simulink model "Shower_model"  (R2020b)
settings: Solver=FixedStepAuto  StartTime=0.0  StopTime=10  RelTol=1e-3
model workspace (MAT data in the model file):
  Idx_1 = [1 1 1 2 2 2 3 3 3]
  Idx_2 = [4 5 6 4 5 6 4 5 6]
  time = [0 0.0625 0.125 0.1875 0.25 0.3125 0.375 0.4375 0.5]
libraries: dspmtrx3 x20, simulink x2
settings Model: ParameterArgumentNames=Idx_1,Idx_2,time  OrderedModelArguments=off  Creator=Deept  LastModifiedBy=Deept
settings DebuggingCC: UnderSpecifiedDimensionMsg=warning

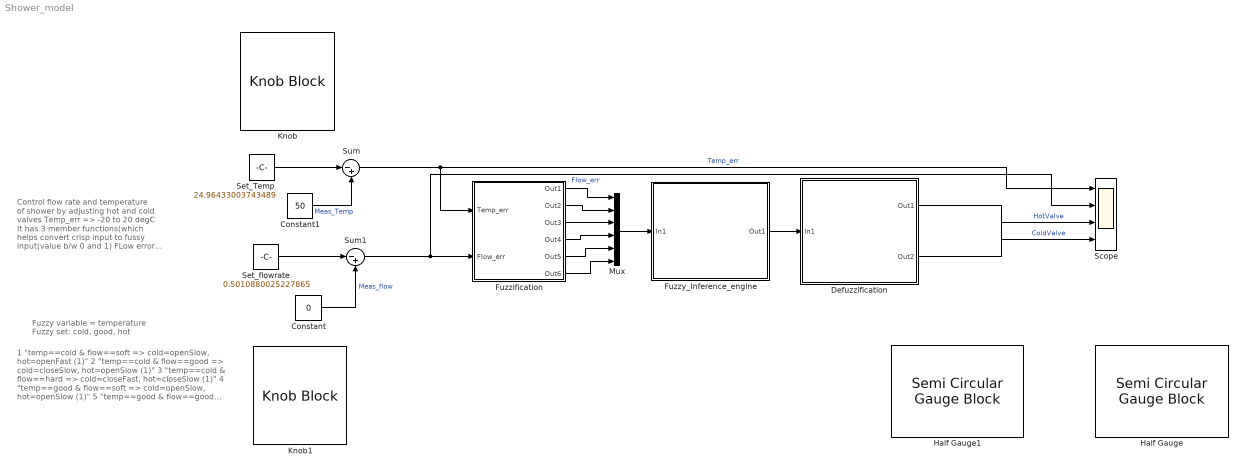
== system Shower_model ==
  note: Fuzzy variable = temperature
      | Fuzzy set: cold, good, hot
  note: 1 "temp==cold & flow==soft => cold=openSlow, hot=openFast (1)"
      | 2 "temp==cold & flow==good => cold=closeSlow, hot=openSlow (1)"
      | 3 "temp==cold & flow==hard => cold=closeFast, hot=closeSlow (1)"
      | 4 "temp==good & flow==soft => cold=openSlow, hot=openSlow (1)"
      | 5 "temp==good & flow==good => cold=steady, hot=steady (1)"
      | 6 "temp==good & flow==hard => cold=closeSlow, hot=closeSlow (1)"
      | 7 "temp==hot & flow==soft => cold=openFast, hot=openSlow (1)"
      | 8 "temp==hot & flow==good => cold=openSlow, hot=closeSlow (1)"
      | 9 "temp==hot & flow==hard => cold=closeSlow, hot=closeFast (1)"
  note: Control flow rate and temperature of shower by adjusting hot and cold valves
      |
      | Temp_err => -20 to 20 degC
      | It has 3 member functions(which helps convert crisp input to fussy input(value b/w 0 and 1)
      | FLow error => -1 to 1
  Constant : Constant  Value=0
  Constant1 : Constant  Value=50
  Defuzzification : Subsystem
  Fuzzification : Subsystem
  Fuzzy_Inference_engine : Subsystem
  Half Gauge : SemiCircularGaugeBlock  LabelPosition=Bottom  ScaleMin=-1  ScaleMax=1
  Half Gauge1 : SemiCircularGaugeBlock  LabelPosition=Bottom  ScaleMin=-1  ScaleMax=1
  Knob : KnobBlock  LabelPosition=Bottom  ScaleMin=20  ScaleMax=30
  Knob1 : KnobBlock  LabelPosition=Bottom  ScaleMax=1
  Mux : Mux  Inputs=6
  Scope : Scope  NumInputPorts=4
  Set_Temp : Constant  Value=24.96433003743489
  Set_flowrate : Constant  Value=0.5010880025227865
  Sum : Sum  Inputs=|-+
  Sum1 : Sum  Inputs=|-+
  wires:
  Set_Temp/1 -> Sum/1
  Set_flowrate/1 -> Sum1/1
  Constant1/1 -> Sum/2  "Meas_Temp"
  Constant/1 -> Sum1/2  "Meas_flow"
  Mux/1 -> Fuzzy_Inference_engine/1(In1)
  Sum/1 -> Fuzzification/1(Temp_err), Scope/1  "Temp_err"
  Sum1/1 -> Fuzzification/2(Flow_err), Scope/2  "Flow_err"
  Fuzzification/1(Out1) -> Mux/1
  Fuzzification/2(Out2) -> Mux/2
  Fuzzification/3(Out3) -> Mux/3
  Fuzzification/4(Out4) -> Mux/4
  Fuzzification/5(Out5) -> Mux/5
  Fuzzification/6(Out6) -> Mux/6
  Fuzzy_Inference_engine/1(Out1) -> Defuzzification/1(In1)
  Defuzzification/1(Out1) -> Scope/4  "ColdValve"
  Defuzzification/2(Out2) -> Scope/3  "HotValve"

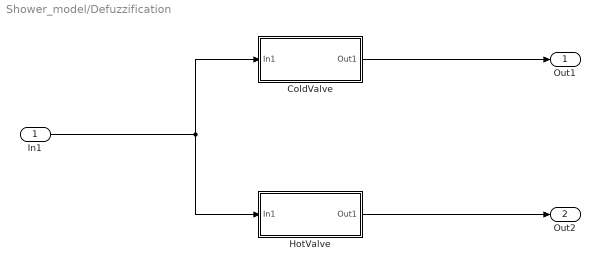
== system Shower_model/Defuzzification ==
  In1 : Inport
  ColdValve : Subsystem
  HotValve : Subsystem
  Out1 : Outport
  Out2 : Outport  Port=2
  wires:
  In1/1 -> ColdValve/1(In1), HotValve/1(In1)
  ColdValve/1(Out1) -> Out1/1
  HotValve/1(Out1) -> Out2/1

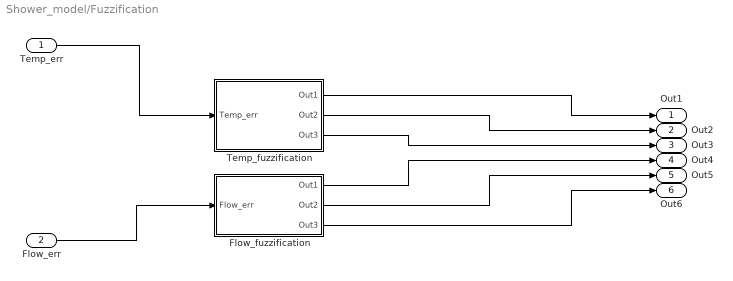
== system Shower_model/Fuzzification ==
  Temp_err : Inport
  Flow_err : Inport  Port=2
  Flow_fuzzification : Subsystem
  Temp_fuzzification : Subsystem
  Out1 : Outport
  Out2 : Outport  Port=2
  Out3 : Outport  Port=3
  Out4 : Outport  Port=4
  Out5 : Outport  Port=5
  Out6 : Outport  Port=6
  wires:
  Temp_err/1 -> Temp_fuzzification/1(Temp_err)
  Flow_fuzzification/1(Out1) -> Out4/1
  Flow_err/1 -> Flow_fuzzification/1(Flow_err)
  Flow_fuzzification/3(Out3) -> Out6/1
  Flow_fuzzification/2(Out2) -> Out5/1
  Temp_fuzzification/1(Out1) -> Out1/1
  Temp_fuzzification/3(Out3) -> Out3/1
  Temp_fuzzification/2(Out2) -> Out2/1

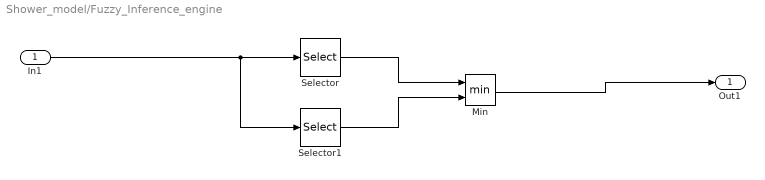
== system Shower_model/Fuzzy_Inference_engine ==
  In1 : Inport
  Min : MinMax  Inputs=2
  Selector : Selector  InputPortWidth=6  IndexOptions=Index vector (dialog)  Indices=idx_1  OutputSizes=1
  Selector1 : Selector  InputPortWidth=6  IndexOptions=Index vector (dialog)  Indices=idx_2  OutputSizes=1
  Out1 : Outport
  wires:
  Min/1 -> Out1/1
  Selector/1 -> Min/1
  Selector1/1 -> Min/2
  In1/1 -> Selector1/1, Selector/1

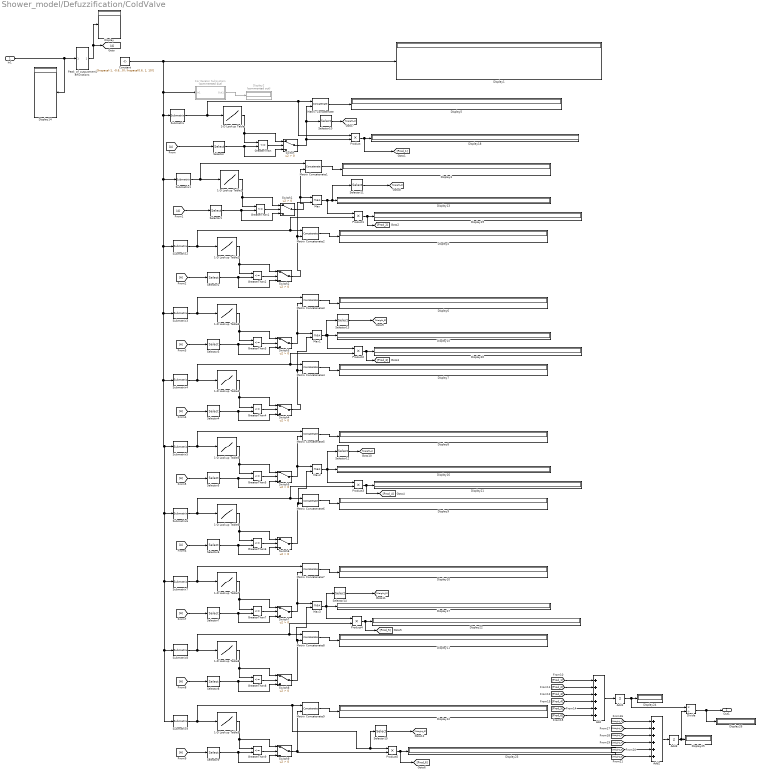
== system Shower_model/Defuzzification/ColdValve ==
  In1 : Inport
  1-D Lookup Table : Lookup_n-D  NumberOfTableDimensions=1  BreakpointsForDimension1=linspace(-1, -0.6, 10)  Table=(linspace(-1, -0.6, 10) + 1) / 0.4  InternalRulePriority=Speed  RndMeth=Simplest  InputSameDT=on
  1-D Lookup Table1 : Lookup_n-D  NumberOfTableDimensions=1  BreakpointsForDimension1=linspace(-0.6, -0.3, 10)  Table=-(linspace(-0.6, -0.3, 10) + 0.3) / 0.3  InternalRulePriority=Speed  RndMeth=Simplest  InputSameDT=on
  1-D Lookup Table2 : Lookup_n-D  NumberOfTableDimensions=1  BreakpointsForDimension1=linspace(-0.6, -0.3, 10)  Table=(linspace(-0.6, -0.3, 10) + 0.6) / 0.3  InternalRulePriority=Speed  RndMeth=Simplest  InputSameDT=on
  1-D Lookup Table3 : Lookup_n-D  NumberOfTableDimensions=1  BreakpointsForDimension1=linspace(-0.3, 0, 10)  Table=-linspace(-0.3, 0, 10) / 0.3  InternalRulePriority=Speed  RndMeth=Simplest  InputSameDT=on
  1-D Lookup Table4 : Lookup_n-D  NumberOfTableDimensions=1  BreakpointsForDimension1=linspace(-0.3, 0, 10)  Table=(linspace(-0.3, 0, 10) + 0.3) / 0.3  InternalRulePriority=Speed  RndMeth=Simplest  InputSameDT=on
  1-D Lookup Table5 : Lookup_n-D  NumberOfTableDimensions=1  BreakpointsForDimension1=linspace(0, 0.3, 10)  Table=-(linspace(0, 0.3, 10) - 0.3) / 0.3  InternalRulePriority=Speed  RndMeth=Simplest  InputSameDT=on
  1-D Lookup Table6 : Lookup_n-D  NumberOfTableDimensions=1  BreakpointsForDimension1=linspace(0, 0.3, 10)  Table=linspace(0, 0.3, 10) / 0.3  InternalRulePriority=Speed  RndMeth=Simplest  InputSameDT=on
  1-D Lookup Table7 : Lookup_n-D  NumberOfTableDimensions=1  BreakpointsForDimension1=linspace(0.3, 0.6, 10)  Table=-(linspace(0.3, 0.6, 10) - 0.6) / 0.3  InternalRulePriority=Speed  RndMeth=Simplest  InputSameDT=on
  1-D Lookup Table8 : Lookup_n-D  NumberOfTableDimensions=1  BreakpointsForDimension1=linspace(0.3, 0.6, 10)  Table=(linspace(0.3, 0.6, 10) - 0.3) / 0.3  InternalRulePriority=Speed  RndMeth=Simplest  InputSameDT=on
  1-D Lookup Table9 : Lookup_n-D  NumberOfTableDimensions=1  BreakpointsForDimension1=linspace(0.6, 1, 10)  Table=-(linspace(0.6, 1, 10) - 1) / 0.4  InternalRulePriority=Speed  RndMeth=Simplest  InputSameDT=on
  Add : Sum  Inputs=++++++
  Add1 : Sum  Inputs=+
  Add2 : Sum  Inputs=++++++
  Add3 : Sum  Inputs=+
  Constant : Constant  Value=[linspace(-1, -0.6, 10); linspace(-0.6, -0.3, 10); linspace(-0.3, 0, 10); linspace(0, 0.3, 10); linspace(0.3, 0.6, 10); linspace(0.6, 1, 10)]
  Display{,1,3..26} (26 alike) : Display
  Display2 : Display  Commented=on
  Divide : Product  Inputs=*/
  For Iterator Subsystem : Subsystem  Commented=on  TreatAsAtomicUnit=on
  GreaterThan{,1..9} (10 alike) : RelationalOperator  Operator=<=  OutDataTypeStr=boolean  RndMeth=Simplest
  Matrix Concatenate{,1..9} (10 alike) : Concatenate  Mode=Multidimensional array  ConcatenateDimension=2
  Max{,1..3} (4 alike) : MinMax  Function=max  Inputs=2
  Peak_of_outputmemberfunctions : Subsystem
  Product{,1..5} (6 alike) : Product
  Selector : Selector  InputPortWidth=5  IndexOptions=Index vector (dialog)  Indices=1  OutputSizes=1
  Selector1 : Selector  InputPortWidth=5  IndexOptions=Index vector (dialog)  Indices=1  OutputSizes=1
  Selector{10..15} (6 alike) : Selector  InputPortWidth=10  IndexOptions=Index vector (dialog)  Indices=[1:9]  OutputSizes=1
  Selector2 : Selector  InputPortWidth=5  IndexOptions=Index vector (dialog)  Indices=2  OutputSizes=1
  Selector3 : Selector  InputPortWidth=5  IndexOptions=Index vector (dialog)  Indices=2  OutputSizes=1
  Selector4 : Selector  InputPortWidth=5  IndexOptions=Index vector (dialog)  Indices=3  OutputSizes=1
  Selector5 : Selector  InputPortWidth=5  IndexOptions=Index vector (dialog)  Indices=3  OutputSizes=1
  Selector6 : Selector  InputPortWidth=5  IndexOptions=Index vector (dialog)  Indices=4  OutputSizes=1
  Selector7 : Selector  InputPortWidth=5  IndexOptions=Index vector (dialog)  Indices=4  OutputSizes=1
  Selector8 : Selector  InputPortWidth=5  IndexOptions=Index vector (dialog)  Indices=5  OutputSizes=1
  Selector9 : Selector  InputPortWidth=5  IndexOptions=Index vector (dialog)  Indices=5  OutputSizes=1
  Submatrix : dspmtrx3/Submatrix  RowSpan=Range of rows  RowStartMode=Index  RowStartIndex=1  RowEndMode=Index  RowEndIndex=1  ColSpan=All columns  ColStartMode=First  ColStartIndex=1  ColEndMode=Last  ColEndIndex=1
  Submatrix1 : dspmtrx3/Submatrix  RowSpan=Range of rows  RowStartMode=Index  RowStartIndex=2  RowEndMode=Index  RowEndIndex=2  ColSpan=All columns  ColStartMode=First  ColStartIndex=1  ColEndMode=Last  ColEndIndex=1
  Submatrix2 : dspmtrx3/Submatrix  RowSpan=Range of rows  RowStartMode=Index  RowStartIndex=2  RowEndMode=Index  RowEndIndex=2  ColSpan=All columns  ColStartMode=First  ColStartIndex=1  ColEndMode=Last  ColEndIndex=1
  Submatrix3 : dspmtrx3/Submatrix  RowSpan=Range of rows  RowStartMode=Index  RowStartIndex=3  RowEndMode=Index  RowEndIndex=3  ColSpan=All columns  ColStartMode=First  ColStartIndex=1  ColEndMode=Last  ColEndIndex=1
  Submatrix4 : dspmtrx3/Submatrix  RowSpan=Range of rows  RowStartMode=Index  RowStartIndex=3  RowEndMode=Index  RowEndIndex=3  ColSpan=All columns  ColStartMode=First  ColStartIndex=1  ColEndMode=Last  ColEndIndex=1
  Submatrix5 : dspmtrx3/Submatrix  RowSpan=Range of rows  RowStartMode=Index  RowStartIndex=4  RowEndMode=Index  RowEndIndex=4  ColSpan=All columns  ColStartMode=First  ColStartIndex=1  ColEndMode=Last  ColEndIndex=1
  Submatrix6 : dspmtrx3/Submatrix  RowSpan=Range of rows  RowStartMode=Index  RowStartIndex=4  RowEndMode=Index  RowEndIndex=4  ColSpan=All columns  ColStartMode=First  ColStartIndex=1  ColEndMode=Last  ColEndIndex=1
  Submatrix7 : dspmtrx3/Submatrix  RowSpan=Range of rows  RowStartMode=Index  RowStartIndex=5  RowEndMode=Index  RowEndIndex=5  ColSpan=All columns  ColStartMode=First  ColStartIndex=1  ColEndMode=Last  ColEndIndex=1
  Submatrix8 : dspmtrx3/Submatrix  RowSpan=Range of rows  RowStartMode=Index  RowStartIndex=5  RowEndMode=Index  RowEndIndex=5  ColSpan=All columns  ColStartMode=First  ColStartIndex=1  ColEndMode=Last  ColEndIndex=1
  Submatrix9 : dspmtrx3/Submatrix  RowSpan=Range of rows  RowStartMode=Index  RowStartIndex=6  RowEndMode=Index  RowEndIndex=6  ColSpan=All columns  ColStartMode=First  ColStartIndex=1  ColEndMode=Last  ColEndIndex=1
  Switch{,1..9} (10 alike) : Switch  Criteria=u2 > Threshold
  Out1 : Outport
  wires:
  In1/1 -> Display14/1, Peak_of_outputmemberfunctions/1(In1)
  Peak_of_outputmemberfunctions/1(Out1) -> [A], Display/1
  For Iterator Subsystem/1(Out1) -> Display2/1
  1-D Lookup Table/1 -> Switch/1, GreaterThan/1
  [A] -> Selector/1
  GreaterThan/1 -> Switch/2
  Selector/1 -> Switch/3, GreaterThan/2
  GreaterThan1/1 -> Switch1/2
  Selector1/1 -> Switch1/3, GreaterThan1/2
  [A] -> Selector1/1
  1-D Lookup Table1/1 -> Switch1/1, GreaterThan1/1
  Switch/1 -> Product/2, Selector10/1, Matrix Concatenate/2
  Matrix Concatenate/1 -> Display5/1
  Submatrix1/1 -> Matrix Concatenate1/1, 1-D Lookup Table1/1
  Switch1/1 -> Matrix Concatenate1/2, Max/1
  Matrix Concatenate1/1 -> Display3/1
  [A] -> Selector2/1
  Switch2/1 -> Max/2, Matrix Concatenate2/2
  GreaterThan2/1 -> Switch2/2
  1-D Lookup Table2/1 -> Switch2/1, GreaterThan2/1
  Selector2/1 -> Switch2/3, GreaterThan2/2
  1-D Lookup Table3/1 -> Switch3/1, GreaterThan3/1
  GreaterThan3/1 -> Switch3/2
  [A] -> Selector3/1
  Selector3/1 -> Switch3/3, GreaterThan3/2
  Matrix Concatenate3/1 -> Display6/1
  Submatrix3/1 -> Matrix Concatenate3/1, 1-D Lookup Table3/1
  Matrix Concatenate4/1 -> Display7/1
  Selector4/1 -> Switch4/3, GreaterThan4/2
  [A] -> Selector4/1
  1-D Lookup Table4/1 -> Switch4/1, GreaterThan4/1
  GreaterThan4/1 -> Switch4/2
  GreaterThan5/1 -> Switch5/2
  Submatrix5/1 -> Matrix Concatenate5/1, 1-D Lookup Table5/1
  1-D Lookup Table5/1 -> Switch5/1, GreaterThan5/1
  Matrix Concatenate5/1 -> Display8/1
  Selector5/1 -> Switch5/3, GreaterThan5/2
  [A] -> Selector5/1
  Matrix Concatenate6/1 -> Display9/1
  [A] -> Selector6/1
  Selector6/1 -> Switch6/3, GreaterThan6/2
  1-D Lookup Table6/1 -> Switch6/1, GreaterThan6/1
  GreaterThan6/1 -> Switch6/2
  1-D Lookup Table7/1 -> Switch7/1, GreaterThan7/1
  GreaterThan7/1 -> Switch7/2
  Submatrix7/1 -> Matrix Concatenate7/1, 1-D Lookup Table7/1
  Selector7/1 -> Switch7/3, GreaterThan7/2
  [A] -> Selector7/1
  Matrix Concatenate7/1 -> Display10/1
  Selector8/1 -> Switch8/3, GreaterThan8/2
  [A] -> Selector8/1
  Matrix Concatenate8/1 -> Display11/1
  GreaterThan8/1 -> Switch8/2
  1-D Lookup Table8/1 -> Switch8/1, GreaterThan8/1
  Constant/1 -> For Iterator Subsystem/1(In1), Submatrix2/1, Submatrix9/1, Submatrix8/1, Submatrix7/1, Submatrix6/1, Submatrix5/1, Submatrix4/1, Submatrix3/1, Submatrix1/1, Submatrix/1, Display1/1
  Selector9/1 -> Switch9/3, GreaterThan9/2
  1-D Lookup Table9/1 -> Switch9/1, GreaterThan9/1
  GreaterThan9/1 -> Switch9/2
  [A] -> Selector9/1
  Matrix Concatenate9/1 -> Display12/1
  Matrix Concatenate2/1 -> Display4/1
  Switch3/1 -> Max1/1, Matrix Concatenate3/2
  Switch4/1 -> Max1/2, Matrix Concatenate4/2
  Switch5/1 -> Max2/1, Matrix Concatenate5/2
  Switch6/1 -> Max2/2, Matrix Concatenate6/2
  Switch8/1 -> Matrix Concatenate8/2, Max3/2
  Switch7/1 -> Max3/1, Matrix Concatenate7/2
  Product/1 -> [Prod_1], Display18/1
  Submatrix2/1 -> Product1/2, Matrix Concatenate2/1, 1-D Lookup Table2/1
  Product1/1 -> [Prod_2], Display19/1
  Max/1 -> Selector11/1, Display13/1, Product1/1
  Max1/1 -> Selector13/1, Product2/1, Display15/1
  Submatrix4/1 -> Product2/2, Matrix Concatenate4/1, 1-D Lookup Table4/1
  Product2/1 -> [Prod_3], Display20/1
  Max2/1 -> Product3/1, Selector12/1, Display16/1
  Product3/1 -> [Prod_4], Display21/1
  Submatrix6/1 -> Product3/2, Matrix Concatenate6/1, 1-D Lookup Table6/1
  Max3/1 -> Selector14/1, Product4/1, Display17/1
  Product4/1 -> [Prod_5], Display22/1
  Submatrix8/1 -> Product4/2, Matrix Concatenate8/1, 1-D Lookup Table8/1
  Submatrix9/1 -> Selector15/1, Product5/1, Matrix Concatenate9/1, 1-D Lookup Table9/1
  Product5/1 -> [Prod_6], Display23/1
  Switch9/1 -> Matrix Concatenate9/2, Product5/2
  [Prod_1] -> Add/1
  [Prod_2] -> Add/2
  [Prod_3] -> Add/3
  [Prod_4] -> Add/4
  [Prod_5] -> Add/5
  [Prod_6] -> Add/6
  Add/1 -> Add1/1
  Add1/1 -> Divide/1, Display24/1
  [Weight_3] -> Add2/3
  [Weight_6] -> Add2/6
  [Weight_1] -> Add2/1
  [Weight_5] -> Add2/5
  [Weight_2] -> Add2/2
  [Weight_4] -> Add2/4
  Add2/1 -> Add3/1
  Add3/1 -> Divide/2, Display25/1
  Submatrix/1 -> Matrix Concatenate/1, Product/1, 1-D Lookup Table/1
  Selector10/1 -> [Weight_1]
  Selector11/1 -> [Weight_2]
  Selector13/1 -> [Weight_3]
  Selector12/1 -> [Weight_4]
  Selector14/1 -> [Weight_5]
  Selector15/1 -> [Weight_6]
  Divide/1 -> Out1/1, Display26/1

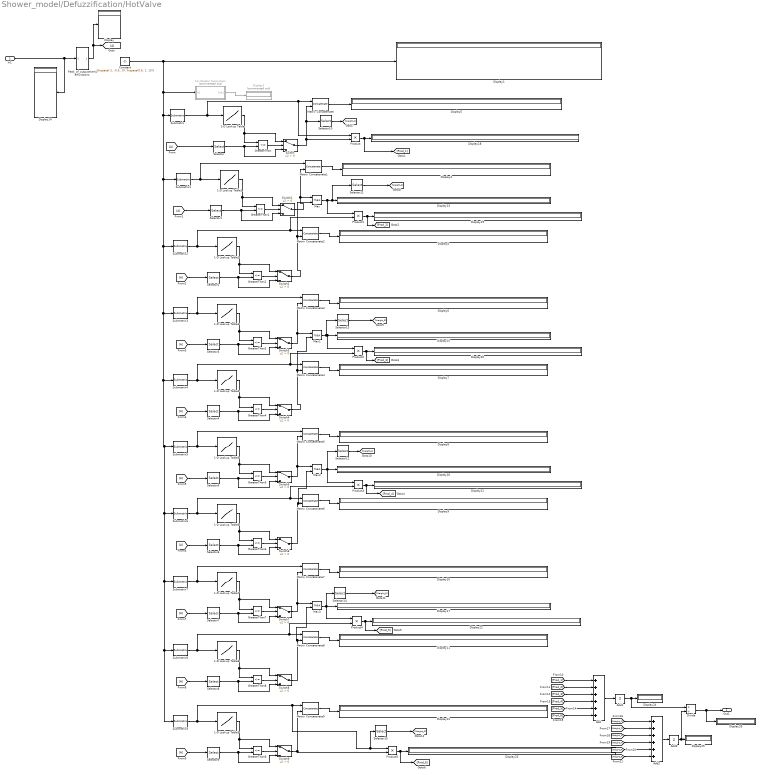
== system Shower_model/Defuzzification/HotValve ==
  In1 : Inport
  1-D Lookup Table : Lookup_n-D  NumberOfTableDimensions=1  BreakpointsForDimension1=linspace(-1, -0.6, 10)  Table=(linspace(-1, -0.6, 10) + 1) / 0.4  InternalRulePriority=Speed  RndMeth=Simplest  InputSameDT=on
  1-D Lookup Table1 : Lookup_n-D  NumberOfTableDimensions=1  BreakpointsForDimension1=linspace(-0.6, -0.3, 10)  Table=-(linspace(-0.6, -0.3, 10) + 0.3) / 0.3  InternalRulePriority=Speed  RndMeth=Simplest  InputSameDT=on
  1-D Lookup Table2 : Lookup_n-D  NumberOfTableDimensions=1  BreakpointsForDimension1=linspace(-0.6, -0.3, 10)  Table=(linspace(-0.6, -0.3, 10) + 0.6) / 0.3  InternalRulePriority=Speed  RndMeth=Simplest  InputSameDT=on
  1-D Lookup Table3 : Lookup_n-D  NumberOfTableDimensions=1  BreakpointsForDimension1=linspace(-0.3, 0, 10)  Table=-linspace(-0.3, 0, 10) / 0.3  InternalRulePriority=Speed  RndMeth=Simplest  InputSameDT=on
  1-D Lookup Table4 : Lookup_n-D  NumberOfTableDimensions=1  BreakpointsForDimension1=linspace(-0.3, 0, 10)  Table=(linspace(-0.3, 0, 10) + 0.3) / 0.3  InternalRulePriority=Speed  RndMeth=Simplest  InputSameDT=on
  1-D Lookup Table5 : Lookup_n-D  NumberOfTableDimensions=1  BreakpointsForDimension1=linspace(0, 0.3, 10)  Table=-(linspace(0, 0.3, 10) - 0.3) / 0.3  InternalRulePriority=Speed  RndMeth=Simplest  InputSameDT=on
  1-D Lookup Table6 : Lookup_n-D  NumberOfTableDimensions=1  BreakpointsForDimension1=linspace(0, 0.3, 10)  Table=linspace(0, 0.3, 10) / 0.3  InternalRulePriority=Speed  RndMeth=Simplest  InputSameDT=on
  1-D Lookup Table7 : Lookup_n-D  NumberOfTableDimensions=1  BreakpointsForDimension1=linspace(0.3, 0.6, 10)  Table=-(linspace(0.3, 0.6, 10) - 0.6) / 0.3  InternalRulePriority=Speed  RndMeth=Simplest  InputSameDT=on
  1-D Lookup Table8 : Lookup_n-D  NumberOfTableDimensions=1  BreakpointsForDimension1=linspace(0.3, 0.6, 10)  Table=(linspace(0.3, 0.6, 10) - 0.3) / 0.3  InternalRulePriority=Speed  RndMeth=Simplest  InputSameDT=on
  1-D Lookup Table9 : Lookup_n-D  NumberOfTableDimensions=1  BreakpointsForDimension1=linspace(0.6, 1, 10)  Table=-(linspace(0.6, 1, 10) - 1) / 0.4  InternalRulePriority=Speed  RndMeth=Simplest  InputSameDT=on
  Add : Sum  Inputs=++++++
  Add1 : Sum  Inputs=+
  Add2 : Sum  Inputs=++++++
  Add3 : Sum  Inputs=+
  Constant : Constant  Value=[linspace(-1, -0.6, 10); linspace(-0.6, -0.3, 10); linspace(-0.3, 0, 10); linspace(0, 0.3, 10); linspace(0.3, 0.6, 10); linspace(0.6, 1, 10)]
  Display{,1,3..26} (26 alike) : Display
  Display2 : Display  Commented=on
  Divide : Product  Inputs=*/
  For Iterator Subsystem : Subsystem  Commented=on  TreatAsAtomicUnit=on
  GreaterThan{,1..9} (10 alike) : RelationalOperator  Operator=<=  OutDataTypeStr=boolean  RndMeth=Simplest
  Matrix Concatenate{,1..9} (10 alike) : Concatenate  Mode=Multidimensional array  ConcatenateDimension=2
  Max{,1..3} (4 alike) : MinMax  Function=max  Inputs=2
  Peak_of_outputmemberfunctions : Subsystem
  Product{,1..5} (6 alike) : Product
  Selector : Selector  InputPortWidth=5  IndexOptions=Index vector (dialog)  Indices=1  OutputSizes=1
  Selector1 : Selector  InputPortWidth=5  IndexOptions=Index vector (dialog)  Indices=1  OutputSizes=1
  Selector{10..15} (6 alike) : Selector  InputPortWidth=10  IndexOptions=Index vector (dialog)  Indices=[1:9]  OutputSizes=1
  Selector2 : Selector  InputPortWidth=5  IndexOptions=Index vector (dialog)  Indices=2  OutputSizes=1
  Selector3 : Selector  InputPortWidth=5  IndexOptions=Index vector (dialog)  Indices=2  OutputSizes=1
  Selector4 : Selector  InputPortWidth=5  IndexOptions=Index vector (dialog)  Indices=3  OutputSizes=1
  Selector5 : Selector  InputPortWidth=5  IndexOptions=Index vector (dialog)  Indices=3  OutputSizes=1
  Selector6 : Selector  InputPortWidth=5  IndexOptions=Index vector (dialog)  Indices=4  OutputSizes=1
  Selector7 : Selector  InputPortWidth=5  IndexOptions=Index vector (dialog)  Indices=4  OutputSizes=1
  Selector8 : Selector  InputPortWidth=5  IndexOptions=Index vector (dialog)  Indices=5  OutputSizes=1
  Selector9 : Selector  InputPortWidth=5  IndexOptions=Index vector (dialog)  Indices=5  OutputSizes=1
  Submatrix : dspmtrx3/Submatrix  RowSpan=Range of rows  RowStartMode=Index  RowStartIndex=1  RowEndMode=Index  RowEndIndex=1  ColSpan=All columns  ColStartMode=First  ColStartIndex=1  ColEndMode=Last  ColEndIndex=1
  Submatrix1 : dspmtrx3/Submatrix  RowSpan=Range of rows  RowStartMode=Index  RowStartIndex=2  RowEndMode=Index  RowEndIndex=2  ColSpan=All columns  ColStartMode=First  ColStartIndex=1  ColEndMode=Last  ColEndIndex=1
  Submatrix2 : dspmtrx3/Submatrix  RowSpan=Range of rows  RowStartMode=Index  RowStartIndex=2  RowEndMode=Index  RowEndIndex=2  ColSpan=All columns  ColStartMode=First  ColStartIndex=1  ColEndMode=Last  ColEndIndex=1
  Submatrix3 : dspmtrx3/Submatrix  RowSpan=Range of rows  RowStartMode=Index  RowStartIndex=3  RowEndMode=Index  RowEndIndex=3  ColSpan=All columns  ColStartMode=First  ColStartIndex=1  ColEndMode=Last  ColEndIndex=1
  Submatrix4 : dspmtrx3/Submatrix  RowSpan=Range of rows  RowStartMode=Index  RowStartIndex=3  RowEndMode=Index  RowEndIndex=3  ColSpan=All columns  ColStartMode=First  ColStartIndex=1  ColEndMode=Last  ColEndIndex=1
  Submatrix5 : dspmtrx3/Submatrix  RowSpan=Range of rows  RowStartMode=Index  RowStartIndex=4  RowEndMode=Index  RowEndIndex=4  ColSpan=All columns  ColStartMode=First  ColStartIndex=1  ColEndMode=Last  ColEndIndex=1
  Submatrix6 : dspmtrx3/Submatrix  RowSpan=Range of rows  RowStartMode=Index  RowStartIndex=4  RowEndMode=Index  RowEndIndex=4  ColSpan=All columns  ColStartMode=First  ColStartIndex=1  ColEndMode=Last  ColEndIndex=1
  Submatrix7 : dspmtrx3/Submatrix  RowSpan=Range of rows  RowStartMode=Index  RowStartIndex=5  RowEndMode=Index  RowEndIndex=5  ColSpan=All columns  ColStartMode=First  ColStartIndex=1  ColEndMode=Last  ColEndIndex=1
  Submatrix8 : dspmtrx3/Submatrix  RowSpan=Range of rows  RowStartMode=Index  RowStartIndex=5  RowEndMode=Index  RowEndIndex=5  ColSpan=All columns  ColStartMode=First  ColStartIndex=1  ColEndMode=Last  ColEndIndex=1
  Submatrix9 : dspmtrx3/Submatrix  RowSpan=Range of rows  RowStartMode=Index  RowStartIndex=6  RowEndMode=Index  RowEndIndex=6  ColSpan=All columns  ColStartMode=First  ColStartIndex=1  ColEndMode=Last  ColEndIndex=1
  Switch{,1..9} (10 alike) : Switch  Criteria=u2 > Threshold
  Out1 : Outport
  wires:
  In1/1 -> Display14/1, Peak_of_outputmemberfunctions/1(In1)
  Peak_of_outputmemberfunctions/1(Out1) -> [A], Display/1
  For Iterator Subsystem/1(Out1) -> Display2/1
  1-D Lookup Table/1 -> Switch/1, GreaterThan/1
  [A] -> Selector/1
  GreaterThan/1 -> Switch/2
  Selector/1 -> Switch/3, GreaterThan/2
  GreaterThan1/1 -> Switch1/2
  Selector1/1 -> Switch1/3, GreaterThan1/2
  [A] -> Selector1/1
  1-D Lookup Table1/1 -> Switch1/1, GreaterThan1/1
  Switch/1 -> Product/2, Selector10/1, Matrix Concatenate/2
  Matrix Concatenate/1 -> Display5/1
  Submatrix1/1 -> Matrix Concatenate1/1, 1-D Lookup Table1/1
  Switch1/1 -> Matrix Concatenate1/2, Max/1
  Matrix Concatenate1/1 -> Display3/1
  [A] -> Selector2/1
  Switch2/1 -> Max/2, Matrix Concatenate2/2
  GreaterThan2/1 -> Switch2/2
  1-D Lookup Table2/1 -> Switch2/1, GreaterThan2/1
  Selector2/1 -> Switch2/3, GreaterThan2/2
  1-D Lookup Table3/1 -> Switch3/1, GreaterThan3/1
  GreaterThan3/1 -> Switch3/2
  [A] -> Selector3/1
  Selector3/1 -> Switch3/3, GreaterThan3/2
  Matrix Concatenate3/1 -> Display6/1
  Submatrix3/1 -> Matrix Concatenate3/1, 1-D Lookup Table3/1
  Matrix Concatenate4/1 -> Display7/1
  Selector4/1 -> Switch4/3, GreaterThan4/2
  [A] -> Selector4/1
  1-D Lookup Table4/1 -> Switch4/1, GreaterThan4/1
  GreaterThan4/1 -> Switch4/2
  GreaterThan5/1 -> Switch5/2
  Submatrix5/1 -> Matrix Concatenate5/1, 1-D Lookup Table5/1
  1-D Lookup Table5/1 -> Switch5/1, GreaterThan5/1
  Matrix Concatenate5/1 -> Display8/1
  Selector5/1 -> Switch5/3, GreaterThan5/2
  [A] -> Selector5/1
  Matrix Concatenate6/1 -> Display9/1
  [A] -> Selector6/1
  Selector6/1 -> Switch6/3, GreaterThan6/2
  1-D Lookup Table6/1 -> Switch6/1, GreaterThan6/1
  GreaterThan6/1 -> Switch6/2
  1-D Lookup Table7/1 -> Switch7/1, GreaterThan7/1
  GreaterThan7/1 -> Switch7/2
  Submatrix7/1 -> Matrix Concatenate7/1, 1-D Lookup Table7/1
  Selector7/1 -> Switch7/3, GreaterThan7/2
  [A] -> Selector7/1
  Matrix Concatenate7/1 -> Display10/1
  Selector8/1 -> Switch8/3, GreaterThan8/2
  [A] -> Selector8/1
  Matrix Concatenate8/1 -> Display11/1
  GreaterThan8/1 -> Switch8/2
  1-D Lookup Table8/1 -> Switch8/1, GreaterThan8/1
  Constant/1 -> For Iterator Subsystem/1(In1), Submatrix2/1, Submatrix9/1, Submatrix8/1, Submatrix7/1, Submatrix6/1, Submatrix5/1, Submatrix4/1, Submatrix3/1, Submatrix1/1, Submatrix/1, Display1/1
  Selector9/1 -> Switch9/3, GreaterThan9/2
  1-D Lookup Table9/1 -> Switch9/1, GreaterThan9/1
  GreaterThan9/1 -> Switch9/2
  [A] -> Selector9/1
  Matrix Concatenate9/1 -> Display12/1
  Matrix Concatenate2/1 -> Display4/1
  Switch3/1 -> Max1/1, Matrix Concatenate3/2
  Switch4/1 -> Max1/2, Matrix Concatenate4/2
  Switch5/1 -> Max2/1, Matrix Concatenate5/2
  Switch6/1 -> Max2/2, Matrix Concatenate6/2
  Switch8/1 -> Matrix Concatenate8/2, Max3/2
  Switch7/1 -> Max3/1, Matrix Concatenate7/2
  Product/1 -> [Prod_1], Display18/1
  Submatrix2/1 -> Product1/2, Matrix Concatenate2/1, 1-D Lookup Table2/1
  Product1/1 -> [Prod_2], Display19/1
  Max/1 -> Selector11/1, Display13/1, Product1/1
  Max1/1 -> Selector13/1, Product2/1, Display15/1
  Submatrix4/1 -> Product2/2, Matrix Concatenate4/1, 1-D Lookup Table4/1
  Product2/1 -> [Prod_3], Display20/1
  Max2/1 -> Product3/1, Selector12/1, Display16/1
  Product3/1 -> [Prod_4], Display21/1
  Submatrix6/1 -> Product3/2, Matrix Concatenate6/1, 1-D Lookup Table6/1
  Max3/1 -> Selector14/1, Product4/1, Display17/1
  Product4/1 -> [Prod_5], Display22/1
  Submatrix8/1 -> Product4/2, Matrix Concatenate8/1, 1-D Lookup Table8/1
  Submatrix9/1 -> Selector15/1, Product5/1, Matrix Concatenate9/1, 1-D Lookup Table9/1
  Product5/1 -> [Prod_6], Display23/1
  Switch9/1 -> Matrix Concatenate9/2, Product5/2
  [Prod_1] -> Add/1
  [Prod_2] -> Add/2
  [Prod_3] -> Add/3
  [Prod_4] -> Add/4
  [Prod_5] -> Add/5
  [Prod_6] -> Add/6
  Add/1 -> Add1/1
  Add1/1 -> Divide/1, Display24/1
  [Weight_3] -> Add2/3
  [Weight_6] -> Add2/6
  [Weight_1] -> Add2/1
  [Weight_5] -> Add2/5
  [Weight_2] -> Add2/2
  [Weight_4] -> Add2/4
  Add2/1 -> Add3/1
  Add3/1 -> Divide/2, Display25/1
  Submatrix/1 -> Matrix Concatenate/1, Product/1, 1-D Lookup Table/1
  Selector10/1 -> [Weight_1]
  Selector11/1 -> [Weight_2]
  Selector13/1 -> [Weight_3]
  Selector12/1 -> [Weight_4]
  Selector14/1 -> [Weight_5]
  Selector15/1 -> [Weight_6]
  Divide/1 -> Out1/1, Display26/1

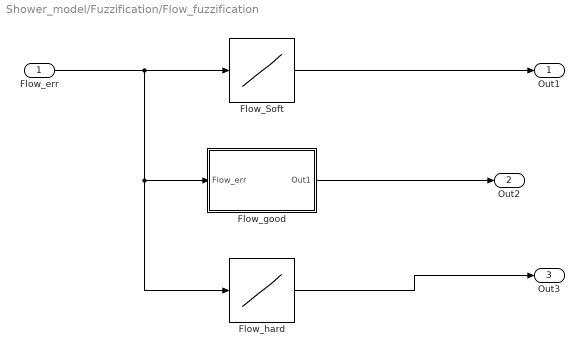
== system Shower_model/Fuzzification/Flow_fuzzification ==
  Flow_err : Inport
  Flow_Soft : Lookup_n-D  NumberOfTableDimensions=1  BreakpointsForDimension1=linspace(-0.8, 0, 10)  Table=(linspace(-0.8, 0, 10)) / (-0.8)  ExtrapMethod=Clip  InternalRulePriority=Speed  RndMeth=Simplest  InputSameDT=on
  Flow_good : Subsystem
  Flow_hard : Lookup_n-D  NumberOfTableDimensions=1  BreakpointsForDimension1=linspace(0, 0.8, 10)  Table=linspace(0, 0.8, 10) / 0.8  ExtrapMethod=Clip  InternalRulePriority=Speed  RndMeth=Simplest  InputSameDT=on
  Out1 : Outport
  Out2 : Outport  Port=2
  Out3 : Outport  Port=3
  wires:
  Flow_err/1 -> Flow_hard/1, Flow_good/1(Flow_err), Flow_Soft/1
  Flow_good/1(Out1) -> Out2/1
  Flow_hard/1 -> Out3/1
  Flow_Soft/1 -> Out1/1

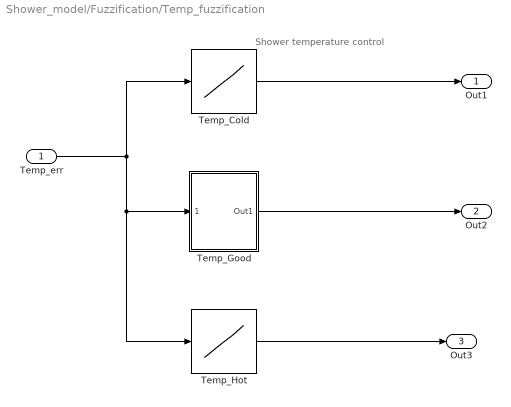
== system Shower_model/Fuzzification/Temp_fuzzification ==
  note: Shower temperature control
  Temp_err : Inport
  Temp_Cold : Lookup_n-D  NumberOfTableDimensions=1  BreakpointsForDimension1=linspace(-15, 0, 10)  Table=(-1 / 15) * linspace(-15, 0, 10)  ExtrapMethod=Clip  InternalRulePriority=Speed  RndMeth=Simplest  InputSameDT=on
  Temp_Good : Subsystem
  Temp_Hot : Lookup_n-D  NumberOfTableDimensions=1  BreakpointsForDimension1=linspace(0, 15, 10)  Table=(1/15) * linspace(0, 15, 10)  ExtrapMethod=Clip  InternalRulePriority=Speed  RndMeth=Simplest  InputSameDT=on
  Out1 : Outport
  Out2 : Outport  Port=2
  Out3 : Outport  Port=3
  wires:
  Temp_Hot/1 -> Out3/1
  Temp_err/1 -> Temp_Hot/1, Temp_Good/1(Temp_err), Temp_Cold/1
  Temp_Good/1(Out1) -> Out2/1
  Temp_Cold/1 -> Out1/1

== system Shower_model/Defuzzification/ColdValve/For Iterator Subsystem ==
  In1 : Inport
  For Iterator : ForIterator  IterationLimit=6
  Selector : Selector  InputPortWidth=6*10  IndexOptions=Index vector (port)  Indices=[1 3]  OutputSizes=1
  Out1 : Outport
  wires:
  For Iterator/1 -> Selector/2
  In1/1 -> Selector/1
  Selector/1 -> Out1/1

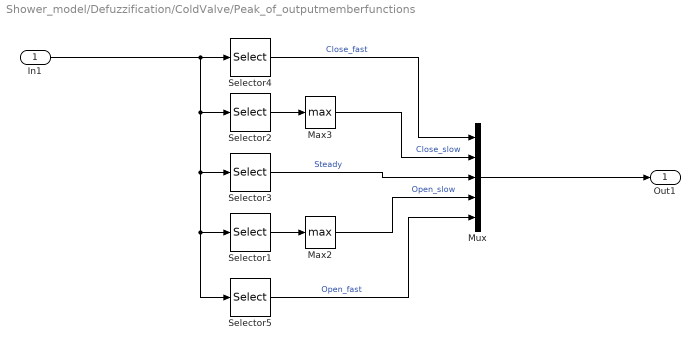
== system Shower_model/Defuzzification/ColdValve/Peak_of_outputmemberfunctions ==
  In1 : Inport
  Max2 : MinMax  Function=max
  Max3 : MinMax  Function=max
  Mux : Mux  Inputs=5
  Selector1 : Selector  InputPortWidth=9  IndexOptions=Index vector (dialog)  Indices=[1 4 8]  OutputSizes=1
  Selector2 : Selector  InputPortWidth=9  IndexOptions=Index vector (dialog)  Indices=[2 6 9]  OutputSizes=1
  Selector3 : Selector  InputPortWidth=9  IndexOptions=Index vector (dialog)  Indices=5  OutputSizes=1
  Selector4 : Selector  InputPortWidth=9  IndexOptions=Index vector (dialog)  Indices=3  OutputSizes=1
  Selector5 : Selector  InputPortWidth=9  IndexOptions=Index vector (dialog)  Indices=7  OutputSizes=1
  Out1 : Outport
  wires:
  Selector4/1 -> Mux/1  "Close_fast"
  Selector1/1 -> Max2/1
  In1/1 -> Selector3/1, Selector1/1, Selector5/1, Selector2/1, Selector4/1
  Max2/1 -> Mux/4  "Open_slow"
  Max3/1 -> Mux/2  "Close_slow"
  Selector5/1 -> Mux/5  "Open_fast"
  Selector3/1 -> Mux/3  "Steady"
  Selector2/1 -> Max3/1
  Mux/1 -> Out1/1

== system Shower_model/Defuzzification/HotValve/For Iterator Subsystem ==
  In1 : Inport
  For Iterator : ForIterator  IterationLimit=6
  Selector : Selector  InputPortWidth=6*10  IndexOptions=Index vector (port)  Indices=[1 3]  OutputSizes=1
  Out1 : Outport
  wires:
  For Iterator/1 -> Selector/2
  In1/1 -> Selector/1
  Selector/1 -> Out1/1

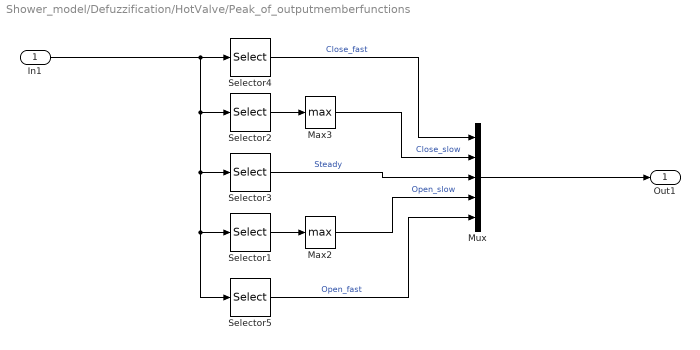
== system Shower_model/Defuzzification/HotValve/Peak_of_outputmemberfunctions ==
  In1 : Inport
  Max2 : MinMax  Function=max
  Max3 : MinMax  Function=max
  Mux : Mux  Inputs=5
  Selector1 : Selector  InputPortWidth=9  IndexOptions=Index vector (dialog)  Indices=[2 4 7]  OutputSizes=1
  Selector2 : Selector  InputPortWidth=9  IndexOptions=Index vector (dialog)  Indices=[3 6 8]  OutputSizes=1
  Selector3 : Selector  InputPortWidth=9  IndexOptions=Index vector (dialog)  Indices=5  OutputSizes=1
  Selector4 : Selector  InputPortWidth=9  IndexOptions=Index vector (dialog)  Indices=9  OutputSizes=1
  Selector5 : Selector  InputPortWidth=9  IndexOptions=Index vector (dialog)  Indices=1  OutputSizes=1
  Out1 : Outport
  wires:
  Selector4/1 -> Mux/1  "Close_fast"
  Selector1/1 -> Max2/1
  In1/1 -> Selector3/1, Selector1/1, Selector5/1, Selector2/1, Selector4/1
  Max2/1 -> Mux/4  "Open_slow"
  Max3/1 -> Mux/2  "Close_slow"
  Selector5/1 -> Mux/5  "Open_fast"
  Selector3/1 -> Mux/3  "Steady"
  Selector2/1 -> Max3/1
  Mux/1 -> Out1/1

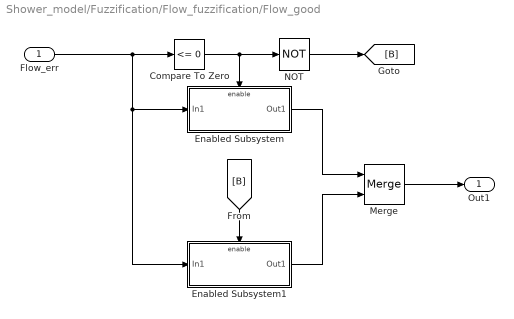
== system Shower_model/Fuzzification/Flow_fuzzification/Flow_good ==
  Flow_err : Inport
  Compare To Zero : simulink/Logic and Bit Operations/Compare To Zero  relop=<=  OutDataTypeStr=boolean
  Enabled Subsystem : Subsystem  TreatAsAtomicUnit=on
  Enabled Subsystem1 : Subsystem  TreatAsAtomicUnit=on
  Merge : Merge
  NOT : Logic  Operator=NOT  IconShape=distinctive  AllPortsSameDT=off  OutDataTypeStr=boolean
  Out1 : Outport
  wires:
  NOT/1 -> [B]
  [B] -> Enabled Subsystem1/Enable
  Compare To Zero/1 -> NOT/1, Enabled Subsystem/Enable
  Flow_err/1 -> Enabled Subsystem1/1(In1), Enabled Subsystem/1(In1), Compare To Zero/1
  Enabled Subsystem/1(Out1) -> Merge/1
  Enabled Subsystem1/1(Out1) -> Merge/2
  Merge/1 -> Out1/1

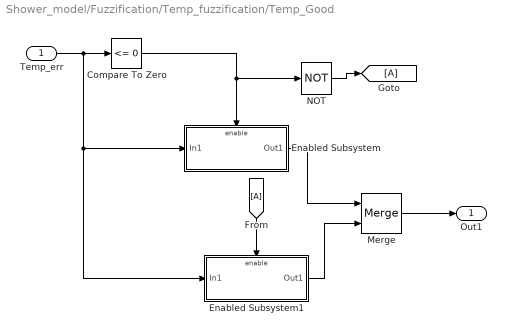
== system Shower_model/Fuzzification/Temp_fuzzification/Temp_Good ==
  Temp_err : Inport
  Compare To Zero : simulink/Logic and Bit Operations/Compare To Zero  relop=<=  OutDataTypeStr=boolean
  Enabled Subsystem : Subsystem  TreatAsAtomicUnit=on
  Enabled Subsystem1 : Subsystem  TreatAsAtomicUnit=on
  Merge : Merge
  NOT : Logic  Operator=NOT  IconShape=distinctive  AllPortsSameDT=off  OutDataTypeStr=boolean
  Out1 : Outport
  wires:
  NOT/1 -> [A]
  Temp_err/1 -> Enabled Subsystem1/1(In1), Enabled Subsystem/1(In1), Compare To Zero/1
  Enabled Subsystem1/1(Out1) -> Merge/2
  Compare To Zero/1 -> Enabled Subsystem/Enable, NOT/1
  Merge/1 -> Out1/1
  [A] -> Enabled Subsystem1/Enable
  Enabled Subsystem/1(Out1) -> Merge/1

== system Shower_model/Fuzzification/Flow_fuzzification/Flow_good/Enabled Subsystem ==
  In1 : Inport
  Enable : EnablePort
  Display : Display
  Flow_soft : Lookup_n-D  NumberOfTableDimensions=1  BreakpointsForDimension1=linspace(-0.4, 0, 10)  Table=(0.40 + linspace(-0.40, 0, 10)) / 0.40  ExtrapMethod=Clip  RndMeth=Simplest  InputSameDT=on
  Out1 : Outport
  wires:
  In1/1 -> Flow_soft/1
  Flow_soft/1 -> Display/1, Out1/1

== system Shower_model/Fuzzification/Flow_fuzzification/Flow_good/Enabled Subsystem1 ==
  In1 : Inport
  Enable : EnablePort
  Flow_hard : Lookup_n-D  NumberOfTableDimensions=1  BreakpointsForDimension1=linspace(0, 0.4, 10)  Table=(0.4 - linspace(0, 0.4, 10)) / 0.4  ExtrapMethod=Clip  InternalRulePriority=Speed  RndMeth=Simplest  InputSameDT=on
  Out1 : Outport
  wires:
  In1/1 -> Flow_hard/1
  Flow_hard/1 -> Out1/1

== system Shower_model/Fuzzification/Temp_fuzzification/Temp_Good/Enabled Subsystem ==
  In1 : Inport
  Enable : EnablePort
  Temp_Good : Lookup_n-D  NumberOfTableDimensions=1  BreakpointsForDimension1=linspace(-10, 0, 10)  Table=(10 + linspace(-10, 0, 10)) / 10  ExtrapMethod=Clip  InternalRulePriority=Speed  RndMeth=Simplest  InputSameDT=on
  Out1 : Outport
  wires:
  In1/1 -> Temp_Good/1
  Temp_Good/1 -> Out1/1

== system Shower_model/Fuzzification/Temp_fuzzification/Temp_Good/Enabled Subsystem1 ==
  In1 : Inport
  Enable : EnablePort
  Temp_Good : Lookup_n-D  NumberOfTableDimensions=1  BreakpointsForDimension1=linspace(0, 10, 10)  Table=(10 - linspace(0, 10, 10)) / 10  ExtrapMethod=Clip  InternalRulePriority=Speed  RndMeth=Simplest  InputSameDT=on
  Out1 : Outport
  wires:
  In1/1 -> Temp_Good/1
  Temp_Good/1 -> Out1/1
